simulink model "automata_learning"  (Simulink 10.3)
settings: Solver=VariableStepAuto  StartTime=0.0  StopTime=10.0  RelTol=1e-3
(part 1 of 2)
settings Model: Creator=diego  LastModifiedBy=diego
settings SolverCC: AlgebraicLoopSolver=Auto
settings DataIOCC: SaveFormat=Dataset  SignalLoggingSaveFormat=Dataset  ReturnWorkspaceOutputs=on
settings OptimizationCC: ExpressionDepthLimit=128  LifeSpan=auto
settings DebuggingCC: UnderspecifiedInitializationDetection=Simplified  MergeDetectMultiDrivingBlocksExec=error  FcnCallInpInsideContextMsg=error  StateNameClashWarn=none  SFUnexpectedBacktrackingDiag=error  SFNoUnconditionalDefaultTransitionDiag=error  SFExecutionAtInitializationDiag=warning  SFMachineParentedDataDiag=error  ArithmeticOperatorsInVariantConditions=error
settings HardwareCC: ProdBitPerPointer=64  ProdBitPerSizeT=64  ProdBitPerPtrDiffT=64  ProdLargestAtomicFloat=Float  ProdIntDivRoundTo=Zero  ProdEndianess=LittleEndian  ProdWordSize=64  ProdHWDeviceType=Intel->x86-64 (Windows64)
settings ModelReferenceCC: PropagateSignalLabelsOutOfModel=on
settings SFSimCC: SimUseLocalCustomCode=on  CustomCodeUndefinedFunction=FilterOut
settings RTWCC: RTWUseLocalCustomCode=on
settings CodeAppCC: StateflowObjectComments=off
settings GRTTargetCC: TargetLangStandard=C99 (ISO)  CombineOutputUpdateFcns=on  GRTInterface=off
settings ConfigComp: CovMetricSettings=dwe  CovSaveCumulativeToWorkspaceVar=off  CovSaveSingleToWorkspaceVar=off  CovExternalEMLEnable=on

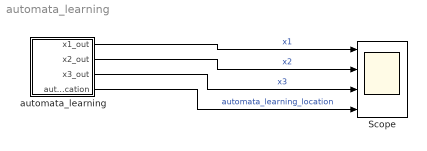
== system automata_learning ==
  Scope : Scope  NumInputPorts=4
  automata_learning : Stateflow chart  TreatAsAtomicUnit=on
  wires:
  automata_learning/1(x1_out) -> Scope/1  "x1"
  automata_learning/2(x2_out) -> Scope/2  "x2"
  automata_learning/3(x3_out) -> Scope/3  "x3"
  automata_learning/4(automata_learning_location) -> Scope/4  "automata_learning_location"
